simulink model "buckConverterVCM"  (R2023a)
settings: Solver=VariableStepAuto  StartTime=0.0  StopTime=.2  MaxStep=.00001  RelTol=1e-3
model workspace (MAT data in the model file):
  C = Simulink.Parameter
  C.Value = 1e-05
  C.DataType = 'auto'
  C.Complexity = 'real'
  C.Dimensions = [1 1]
  L = Simulink.Parameter
  L.Value = 0.00022
  L.DataType = 'auto'
  L.Complexity = 'real'
  L.Dimensions = [1 1]
  R = Simulink.Parameter
  R.Value = 5
  R.DataType = 'auto'
  R.Complexity = 'real'
  R.Dimensions = [1 1]
  Vin = Simulink.Parameter
  Vin.Value = 48
  Vin.DataType = 'auto'
  Vin.Complexity = 'real'
  Vin.Dimensions = [1 1]
values from neighbouring files (symbols this model uses):
  C = 5*10^-4    (= 0.0005)    [parameters.m]
  L = 220*10^-6    (= 0.00022)    [parameters.m]
  R = 5    [parameters.m]
  Vin = 48    [parameters.m]
libraries: spsSeriesRLCBranchLib x6, spsControlledVoltageSourceLib x1, spsCurrentMeasurementLib x1, spsDiodeLib x1, spsIdealSwitchLib x1, spsMosfetLib x1, spsVoltageMeasurementLib x1, spspowerguiLib x1
settings Model: Creator=User  LastModifiedBy=User
settings DebuggingCC: UnconnectedInputMsg=warning  UnconnectedOutputMsg=warning  UnconnectedLineMsg=warning
settings ModelReferenceCC: EnableRefExpFcnMdlSchedulingChecks=on
settings RTWCC: DLArmComputeVersion=19.05

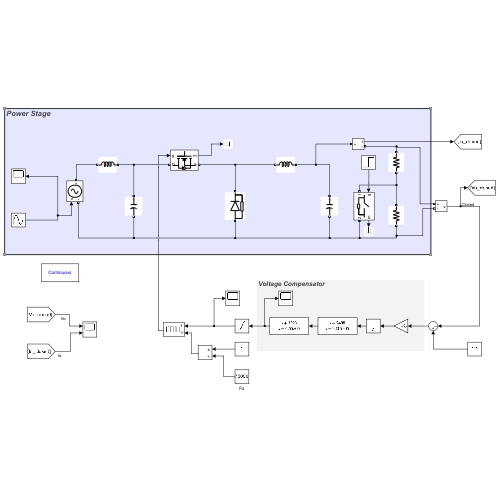
[thumbnail: Simulink's stored preview of the top-level diagram]
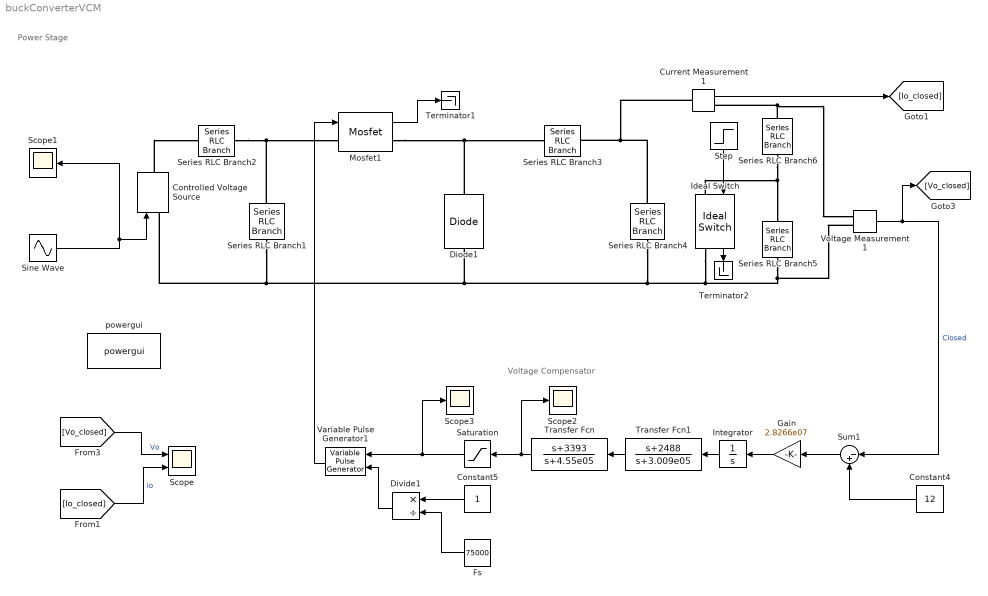
== system buckConverterVCM ==
  note: Voltage Compensator
  note: Power Stage
  Constant4 : Constant  Value=12
  Constant5 : Constant
  Controlled Voltage Source : spsControlledVoltageSourceLib/Controlled Voltage Source  Initialize=on  Source_Type=AC  Amplitude=0  Phase=0  Frequency=0  Measurements=None
  Current Measurement1 : spsCurrentMeasurementLib/Current Measurement  PhasorSimulation=off  OutputType=Complex  PSBequivalent=0
  Diode1 : spsDiodeLib/Diode  Ron=0.001  Lon=0  Vf=0.8  IC=0  UseSnubber=0  Rs=500  Cs=250e-9  Measurements=off
  Divide1 : Product  Inputs=*/
  Fs : Constant  Value=75000
  Gain : Gain  Gain=2.8266e07
  Ideal Switch : spsIdealSwitchLib/Ideal Switch  Ron=0.001  Lon=0  IC=0  Rs=1e5  Cs=inf  Measurements=on
  Integrator : Integrator
  Mosfet1 : spsMosfetLib/Mosfet  Ron=0.1  Lon=0  Rd=0.01  Vfd=0  IC=0  Rs=1e5  Cs=inf  Measurements=on
  Saturation : Saturate  UpperLimit=1  LowerLimit=0
  Scope : Scope  NumInputPorts=2
  Scope1 : Scope
  Scope2 : Scope
  Scope3 : Scope
  Series RLC Branch1 : spsSeriesRLCBranchLib/Series RLC Branch  LConnTagsString=__new0  RConnTagsString=__new0  BranchType=C  Resistance=1  Inductance=1e-3  SetiL0=off  InitialCurrent=0  Capacitance=C  Setx0=off  InitialVoltage=0  Measurements=None
  Series RLC Branch2 : spsSeriesRLCBranchLib/Series RLC Branch  LConnTagsString=__new0  RConnTagsString=__new0  BranchType=L  Resistance=1  Inductance=L  SetiL0=off  InitialCurrent=0  Capacitance=1e-6  Setx0=off  InitialVoltage=0  Measurements=None
  Series RLC Branch3 : spsSeriesRLCBranchLib/Series RLC Branch  LConnTagsString=__new0  RConnTagsString=__new0  BranchType=L  Resistance=1  Inductance=L  SetiL0=off  InitialCurrent=0  Capacitance=1e-6  Setx0=off  InitialVoltage=0  Measurements=None
  Series RLC Branch4 : spsSeriesRLCBranchLib/Series RLC Branch  LConnTagsString=__new0  RConnTagsString=__new0  BranchType=C  Resistance=1  Inductance=1e-3  SetiL0=off  InitialCurrent=0  Capacitance=C  Setx0=off  InitialVoltage=0  Measurements=None
  Series RLC Branch5 : spsSeriesRLCBranchLib/Series RLC Branch  LConnTagsString=__new0  RConnTagsString=__new0  BranchType=R  Resistance=R  Inductance=1e-3  SetiL0=off  InitialCurrent=0  Capacitance=1e-6  Setx0=off  InitialVoltage=0  Measurements=None
  Series RLC Branch6 : spsSeriesRLCBranchLib/Series RLC Branch  LConnTagsString=__new0  RConnTagsString=__new0  BranchType=R  Resistance=R  Inductance=1e-3  SetiL0=off  InitialCurrent=0  Capacitance=1e-6  Setx0=off  InitialVoltage=0  Measurements=None
  Sine Wave : Sin  Amplitude=2  Bias=Vin  Frequency=2*pi*100  SampleTime=0
  Step : Step  Time=.15  SampleTime=0
  Sum1 : Sum  Inputs=|-+
  Terminator1 : Terminator
  Terminator2 : Terminator
  Transfer Fcn : TransferFcn  Numerator=[1 3393]  Denominator=[1 4.55e05]
  Transfer Fcn1 : TransferFcn  Numerator=[1 2488]  Denominator=[1 3.009e05]
  Variable Pulse Generator1 : VariablePulseGenerator  AllowZeroPulseWidth=on  SampleTime=0.1
  Voltage Measurement1 : spsVoltageMeasurementLib/Voltage Measurement  PhasorSimulation=off  OutputType=Complex  PSBequivalent=0
  powergui : spspowerguiLib/powergui  Priority=1  SimulationMode=Continuous  SampleTime=50e-6  frequency=60  Iterations=50  frequencyindice=0  Pbase=100e6  ErrMax=1e-4  UnitsV=kV  UnitsW=MW  buscounter=0  FunctionMessages=off  echomessages=off  EnableUseOfTLC=off  CurrentSourceSwitches=off  DisableSnubberDevices=off  DisableRonSwitches=off  DisableVfSwitches=off  DisplayEquations=off  AutomaticDiscreteSolvers=off  SolverType=Tustin/Backward Euler (TBE)  Interpol=off  ExternalGateDelay=off  methode=off  Ts=100  x0status=blocks  SPID=on  SwTol=0  HookPort=off  NonlinearTolerance=1e-4  nMaxIteration=100  ContinueOnMaxIteration=off  RestoreLinks=warning  ResistiveCurrentMeasurement=off  Frange=[0:2:500]  Ylog=off  Xlog=on  ShowGrid=off  save=off  variable=ZData  structure=0  ZoomFFT=off  StartTime=0.0  cycles=1  DisplayStyle=1  fundamental=60  FreqAxis=off  MaxFrequency=1000  frequencyindicesteady=1  RmsSteady=1  display=off
  wires:
  Mosfet1/1 -> Terminator1/1
  Voltage Measurement1/1 -> [Vo_closed], Sum1/1  "Closed"
  Sum1/1 -> Gain/1
  Transfer Fcn/1 -> Scope2/1, Saturation/1
  Constant5/1 -> Divide1/1
  Fs/1 -> Divide1/2
  Variable Pulse Generator1/1 -> Mosfet1/1
  Saturation/1 -> Scope3/1, Variable Pulse Generator1/1
  Transfer Fcn1/1 -> Transfer Fcn/1
  Gain/1 -> Integrator/1
  Integrator/1 -> Transfer Fcn1/1
  Ideal Switch/1 -> Terminator2/1
  Step/1 -> Ideal Switch/1
  Current Measurement1/1 -> [Io_closed]
  [Io_closed] -> Scope/2  "Io"
  [Vo_closed] -> Scope/1  "Vo"
  Divide1/1 -> Variable Pulse Generator1/2
  Constant4/1 -> Sum1/2
  Sine Wave/1 -> Scope1/1, Controlled Voltage Source/1
  connections:
  Series RLC Branch5/RConn1 -- Ideal Switch/RConn1 -- Series RLC Branch1/RConn1 -- Controlled Voltage Source/LConn1 -- Diode1/LConn1 -- Series RLC Branch4/RConn1 -- Voltage Measurement1/LConn2
  Diode1/RConn1 -- Series RLC Branch3/LConn1 -- Mosfet1/RConn1
  Series RLC Branch3/RConn1 -- Series RLC Branch4/LConn1 -- Current Measurement1/LConn1
  Series RLC Branch2/RConn1 -- Series RLC Branch1/LConn1 -- Mosfet1/LConn1
  Ideal Switch/LConn1 -- Series RLC Branch5/LConn1 -- Series RLC Branch6/RConn1
  Current Measurement1/RConn1 -- Voltage Measurement1/LConn1 -- Series RLC Branch6/LConn1
  Controlled Voltage Source/RConn1 -- Series RLC Branch2/LConn1
